simulink model "SIMILACION"  (R2021b)
settings: Solver=VariableStepAuto  StartTime=0.0  StopTime=100  MaxStep=0.001  MinStep=0.0001  RelTol=1e-3
undefined symbols (not defined in the file): C1, L1, L2
libraries: spsSeriesRLCBranchLib x17, spsVoltageMeasurementLib x15, spsParallelRLCBranchLib x13, spsGroundLib x6, spsControlledVoltageSourceLib x3, cstblocks x1, spspowerguiLib x1
settings Model: Creator=Roberto  LastModifiedBy=Roberto

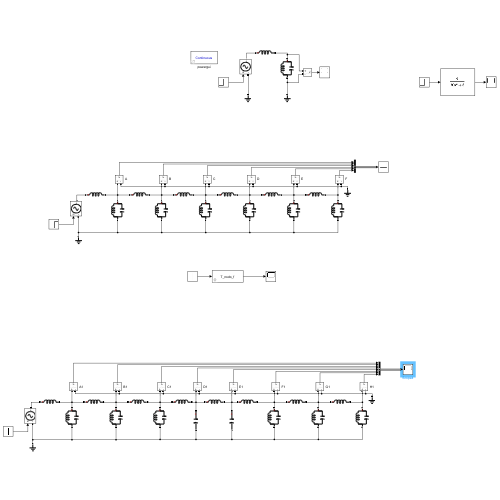
[thumbnail: Simulink's stored preview of the top-level diagram]
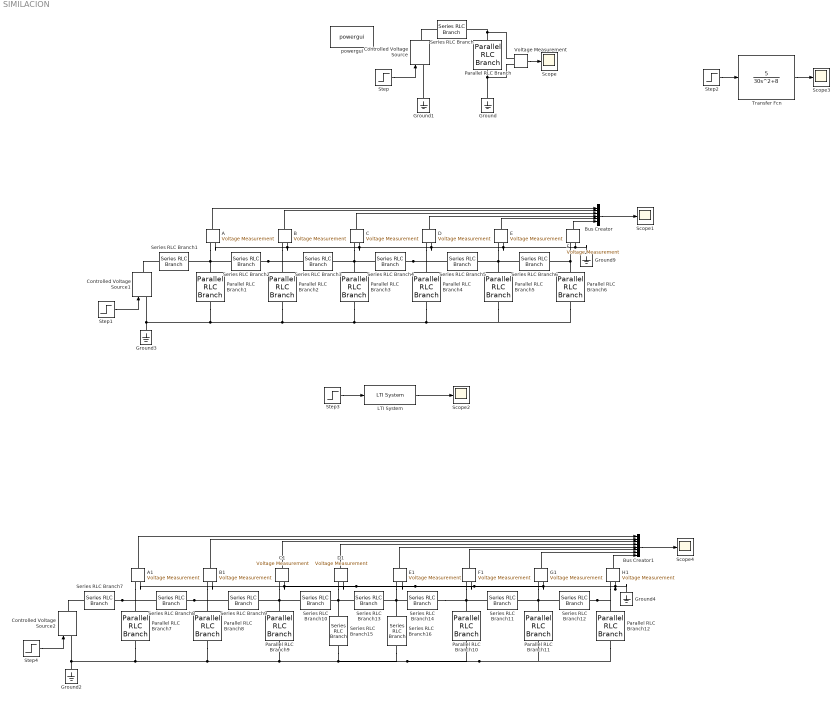
== system SIMILACION ==
  A : spsVoltageMeasurementLib/Voltage Measurement  PhasorSimulation=off  OutputType=Complex  PSBequivalent=0
  A1 : spsVoltageMeasurementLib/Voltage Measurement  PhasorSimulation=off  OutputType=Complex  PSBequivalent=0
  B : spsVoltageMeasurementLib/Voltage Measurement  PhasorSimulation=off  OutputType=Complex  PSBequivalent=0
  B1 : spsVoltageMeasurementLib/Voltage Measurement  PhasorSimulation=off  OutputType=Complex  PSBequivalent=0
  Bus Creator : BusCreator  Inputs=6
  Bus Creator1 : BusCreator  Inputs=8
  C : spsVoltageMeasurementLib/Voltage Measurement  PhasorSimulation=off  OutputType=Complex  PSBequivalent=0
  C1 : spsVoltageMeasurementLib/Voltage Measurement  PhasorSimulation=off  OutputType=Complex  PSBequivalent=0
  Controlled Voltage Source : spsControlledVoltageSourceLib/Controlled Voltage Source  Initialize=on  Source_Type=AC  Amplitude=0  Phase=0  Frequency=0  Measurements=None
  Controlled Voltage Source1 : spsControlledVoltageSourceLib/Controlled Voltage Source  Initialize=on  Source_Type=AC  Amplitude=0  Phase=0  Frequency=0  Measurements=None
  Controlled Voltage Source2 : spsControlledVoltageSourceLib/Controlled Voltage Source  Initialize=on  Source_Type=AC  Amplitude=0  Phase=0  Frequency=0  Measurements=None
  D : spsVoltageMeasurementLib/Voltage Measurement  PhasorSimulation=off  OutputType=Complex  PSBequivalent=0
  D1 : spsVoltageMeasurementLib/Voltage Measurement  PhasorSimulation=off  OutputType=Complex  PSBequivalent=0
  E : spsVoltageMeasurementLib/Voltage Measurement  PhasorSimulation=off  OutputType=Complex  PSBequivalent=0
  E1 : spsVoltageMeasurementLib/Voltage Measurement  PhasorSimulation=off  OutputType=Complex  PSBequivalent=0
  F : spsVoltageMeasurementLib/Voltage Measurement  PhasorSimulation=off  OutputType=Complex  PSBequivalent=0
  F1 : spsVoltageMeasurementLib/Voltage Measurement  PhasorSimulation=off  OutputType=Complex  PSBequivalent=0
  G1 : spsVoltageMeasurementLib/Voltage Measurement  PhasorSimulation=off  OutputType=Complex  PSBequivalent=0
  Ground{,1..4,9} (6 alike) : spsGroundLib/Ground  LConnTagsString=a
  H1 : spsVoltageMeasurementLib/Voltage Measurement  PhasorSimulation=off  OutputType=Complex  PSBequivalent=0
  LTI System : cstblocks/LTI System  sys=T_nodo_f  IC=[]
  Parallel RLC Branch{,1..12} (13 alike) : spsParallelRLCBranchLib/Parallel RLC Branch  LConnTagsString=a  RConnTagsString=__new0  BranchType=LC  Resistance=1  Inductance=L2  SetiL0=off  InitialCurrent=0  Capacitance=C1  Setx0=off  InitialVoltage=0  Measurements=None
  Scope{,1..4} (5 alike) : Scope
  Series RLC Branch{,1..14} (15 alike) : spsSeriesRLCBranchLib/Series RLC Branch  LConnTagsString=__new0  RConnTagsString=__new0  BranchType=L  Resistance=1  Inductance=L1  SetiL0=off  InitialCurrent=0  Capacitance=1e-6  Setx0=off  InitialVoltage=0  Measurements=None
  Series RLC Branch15 : spsSeriesRLCBranchLib/Series RLC Branch  LConnTagsString=__new0  RConnTagsString=__new0  BranchType=C  Resistance=1  Inductance=L1  SetiL0=off  InitialCurrent=0  Capacitance=C1  Setx0=off  InitialVoltage=0  Measurements=None
  Series RLC Branch16 : spsSeriesRLCBranchLib/Series RLC Branch  LConnTagsString=__new0  RConnTagsString=__new0  BranchType=C  Resistance=1  Inductance=L1  SetiL0=off  InitialCurrent=0  Capacitance=C1  Setx0=off  InitialVoltage=0  Measurements=None
  Step{,1..4} (5 alike) : Step  Time=0  SampleTime=0
  Transfer Fcn : TransferFcn  Numerator=[5]  Denominator=[30 0 8]
  Voltage Measurement : spsVoltageMeasurementLib/Voltage Measurement  PhasorSimulation=off  OutputType=Complex  PSBequivalent=0
  powergui : spspowerguiLib/powergui  Priority=1  SimulationMode=Continuous  SampleTime=50e-6  frequency=60  Iterations=50  frequencyindice=0  Pbase=100e6  ErrMax=1e-4  UnitsV=kV  UnitsW=MW  buscounter=0  FunctionMessages=off  echomessages=off  EnableUseOfTLC=off  CurrentSourceSwitches=off  DisableSnubberDevices=off  DisableRonSwitches=off  DisableVfSwitches=off  DisplayEquations=off  AutomaticDiscreteSolvers=off  SolverType=Tustin/Backward Euler (TBE)  Interpol=off  ExternalGateDelay=off  methode=off  Ts=100  x0status=blocks  SPID=on  SwTol=0  HookPort=off  NonlinearTolerance=1e-4  nMaxIteration=100  ContinueOnMaxIteration=off  RestoreLinks=warning  ResistiveCurrentMeasurement=off  Frange=[0:2:500]  Ylog=off  Xlog=on  ShowGrid=off  save=off  variable=ZData  structure=0  ZoomFFT=off  StartTime=0.0  cycles=1  DisplayStyle=1  fundamental=60  FreqAxis=off  MaxFrequency=1000  frequencyindicesteady=1  RmsSteady=1  display=off
  wires:
  Step/1 -> Controlled Voltage Source/1
  Voltage Measurement/1 -> Scope/1
  Step1/1 -> Controlled Voltage Source1/1
  Bus Creator/1 -> Scope1/1
  F/1 -> Bus Creator/6
  E/1 -> Bus Creator/5
  D/1 -> Bus Creator/4
  C/1 -> Bus Creator/3
  B/1 -> Bus Creator/2
  A/1 -> Bus Creator/1
  Step2/1 -> Transfer Fcn/1
  Transfer Fcn/1 -> Scope3/1
  Step3/1 -> LTI System/1
  LTI System/1 -> Scope2/1
  Step4/1 -> Controlled Voltage Source2/1
  Bus Creator1/1 -> Scope4/1
  H1/1 -> Bus Creator1/8
  F1/1 -> Bus Creator1/6
  G1/1 -> Bus Creator1/7
  E1/1 -> Bus Creator1/5
  D1/1 -> Bus Creator1/4
  C1/1 -> Bus Creator1/3
  B1/1 -> Bus Creator1/2
  A1/1 -> Bus Creator1/1
  connections:
  Parallel RLC Branch/LConn1 -- Voltage Measurement/LConn1 -- Series RLC Branch/RConn1
  Ground/LConn1 -- Voltage Measurement/LConn2 -- Parallel RLC Branch/RConn1
  Controlled Voltage Source/RConn1 -- Series RLC Branch/LConn1
  Ground1/LConn1 -- Controlled Voltage Source/LConn1
  Parallel RLC Branch1/LConn1 -- Series RLC Branch2/LConn1 -- A/LConn1 -- Series RLC Branch1/RConn1
  Controlled Voltage Source1/RConn1 -- Series RLC Branch1/LConn1
  Ground3/LConn1 -- Parallel RLC Branch5/RConn1 -- Parallel RLC Branch6/RConn1 -- Parallel RLC Branch4/RConn1 -- Parallel RLC Branch3/RConn1 -- Parallel RLC Branch2/RConn1 -- Parallel RLC Branch1/RConn1 -- Controlled Voltage Source1/LConn1
  Series RLC Branch2/RConn1 -- Series RLC Branch3/LConn1 -- Parallel RLC Branch2/LConn1 -- B/LConn1
  C/LConn1 -- Series RLC Branch4/LConn1 -- Series RLC Branch3/RConn1 -- Parallel RLC Branch3/LConn1
  Series RLC Branch4/RConn1 -- Series RLC Branch5/LConn1 -- Parallel RLC Branch4/LConn1 -- D/LConn1
  E/LConn1 -- Series RLC Branch6/LConn1 -- Series RLC Branch5/RConn1 -- Parallel RLC Branch5/LConn1
  F/LConn1 -- Parallel RLC Branch6/LConn1 -- Series RLC Branch6/RConn1
  A/LConn2 -- B/LConn2 -- C/LConn2 -- E/LConn2 -- Ground9/LConn1 -- F/LConn2 -- D/LConn2
  Parallel RLC Branch8/RConn1 -- Series RLC Branch16/RConn1 -- Parallel RLC Branch12/RConn1 -- Parallel RLC Branch11/RConn1 -- Parallel RLC Branch10/RConn1 -- Series RLC Branch15/RConn1 -- Parallel RLC Branch9/RConn1 -- Parallel RLC Branch7/RConn1 -- Controlled Voltage Source2/LConn1 -- Ground2/LConn1
  Series RLC Branch8/RConn1 -- Series RLC Branch9/LConn1 -- Parallel RLC Branch8/LConn1 -- B1/LConn1
  Series RLC Branch7/RConn1 -- Series RLC Branch8/LConn1 -- Parallel RLC Branch7/LConn1 -- A1/LConn1
  Series RLC Branch12/RConn1 -- H1/LConn1 -- Parallel RLC Branch12/LConn1
  F1/LConn1 -- Series RLC Branch14/RConn1 -- Series RLC Branch11/LConn1 -- Parallel RLC Branch10/LConn1
  G1/LConn1 -- Series RLC Branch12/LConn1 -- Series RLC Branch11/RConn1 -- Parallel RLC Branch11/LConn1
  C1/LConn1 -- Series RLC Branch10/LConn1 -- Series RLC Branch9/RConn1 -- Parallel RLC Branch9/LConn1
  Controlled Voltage Source2/RConn1 -- Series RLC Branch7/LConn1
  H1/LConn2 -- F1/LConn2 -- B1/LConn2 -- A1/LConn2 -- C1/LConn2 -- D1/LConn2 -- E1/LConn2 -- G1/LConn2 -- Ground4/LConn1
  Series RLC Branch14/LConn1 -- E1/LConn1 -- Series RLC Branch16/LConn1 -- Series RLC Branch13/RConn1
  Series RLC Branch13/LConn1 -- D1/LConn1 -- Series RLC Branch15/LConn1 -- Series RLC Branch10/RConn1
